simulink model "z_create_signal"  (R2025b)
settings: Solver=FixedStepAuto  StartTime=0.0  StopTime=0.2  FixedStep=1e-7  RelTol=1e-3
settings Model: Creator=daniel  LastModifiedBy=daniel

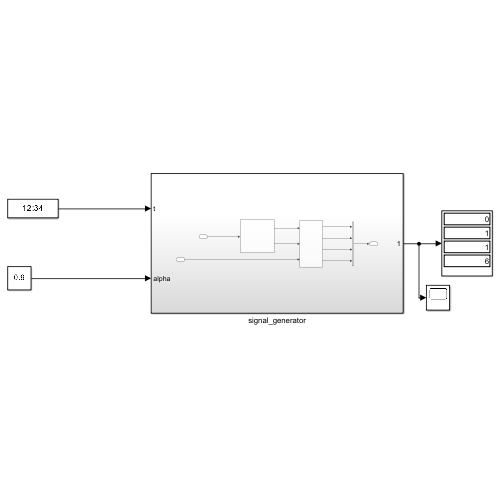
[thumbnail: Simulink's stored preview of the top-level diagram]
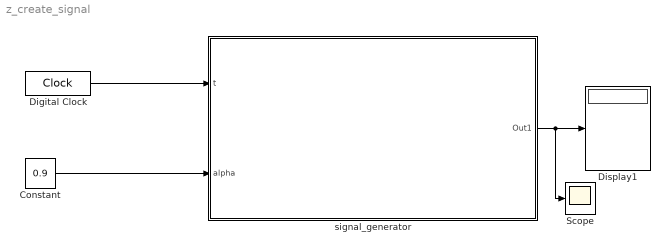
== system z_create_signal ==
  Constant : Constant  Value=0.9
  Digital Clock : DigitalClock  SampleTime=1e-7
  Display1 : Display
  Scope : Scope
      settings: ActiveDisplayYMinimum=-24.748928156893  ActiveDisplayYMaximum=53.111988858956792
  signal_generator : Subsystem
  wires:
  signal_generator/1(Out1) -> Display1/1, Scope/1
  Constant/1 -> signal_generator/2(alpha)
  Digital Clock/1 -> signal_generator/1(t)

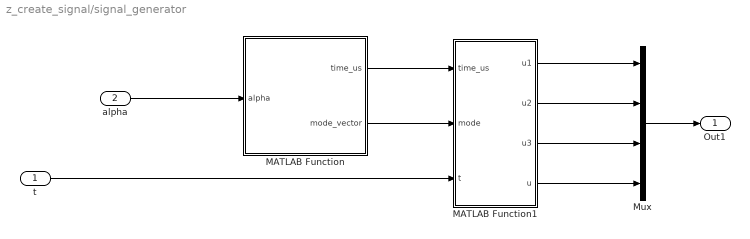
== system z_create_signal/signal_generator ==
  t : Inport
  alpha : Inport  Port=2
  MATLAB Function : MATLAB Function  TreatAsAtomicUnit=on
  MATLAB Function1 : MATLAB Function  TreatAsAtomicUnit=on
  Mux : Mux
  Out1 : Outport
  wires:
  MATLAB Function/2(mode_vector) -> MATLAB Function1/2(mode)
  MATLAB Function/1(time_us) -> MATLAB Function1/1(time_us)
  alpha/1 -> MATLAB Function/1(alpha)
  Mux/1 -> Out1/1
  t/1 -> MATLAB Function1/3(t)
  MATLAB Function1/4(u) -> Mux/4
  MATLAB Function1/1(u1) -> Mux/1
  MATLAB Function1/2(u2) -> Mux/2
  MATLAB Function1/3(u3) -> Mux/3

== matlab function z_create_signal/signal_generator/MATLAB Function1 ==
  data: time_us input; u1 output; mode input; t input; u2 output; u3 output; u output
function [u1, u2, u3, u] = generate_signal(time_us, mode, t)

    [u1, u2, u3, u] = signal_generate(time_us, mode, t);

== matlab function z_create_signal/signal_generator/MATLAB Function ==
  data: alpha input; time_us output; mode_vector output
function [time_us, mode_vector] = fcn(alpha)
    [time_us, mode_vector] = signal_create(alpha);
